simulink model "precompensationVSintegrator"  (R2018b)
settings: Solver=VariableStepAuto  StartTime=0.0  StopTime=2  RelTol=1e-3
values from neighbouring files (symbols this model uses):
  A = [-(bm*(n^2) + bg)/(Jm*(n^2) + Jg) Kt*n/(Jm*(n^2) + Jg) ... (first row only)    [DC_motor_geared_integral_discrete_sysid23.m]    (also in DC_motor_geared_lqr_discrete_sysid23.m; finalScript.m; finalScriptV2.m; precompensatorVSintegrator.m)
  B = [0 ... (first row only)    [DC_motor_geared_integral_discrete_sysid23.m]    (also in DC_motor_geared_lqr_discrete_sysid23.m; finalScript.m; finalScriptV2.m; precompensatorVSintegrator.m)
  Kc = lqr(sysd,Q,R)    [DC_motor_geared_lqr_discrete_sysid23.m]    (also in precompensatorVSintegrator.m = lqr(sysc,Q,R))
  Kdi = dlqr(Ad,Bd,Q,R)    [DC_motor_geared_integral_discrete_sysid23.m]    (also in finalScript.m; finalScriptV2.m)
  Nbar = rscale(sys_ss,Kc)    [DC_motor_geared_lqr_discrete_sysid23.m]    (also in precompensatorVSintegrator.m; rscale.m = Nu + K*Nx)
  Tsc = 1/20000    (= 5e-05)    [DC_motor_geared_integral_discrete_sysid23.m]    (also in DC_motor_geared_lqr_discrete_sysid23.m = 1e-05; finalScript.m; finalScriptV2.m = 0.001)
undefined symbols (not defined in the file or in its folder): DiscIntNeverNeededParam
libraries: pePwmGenerator x2
settings Model: Creator=Roberto  LastModifiedBy=Roberto

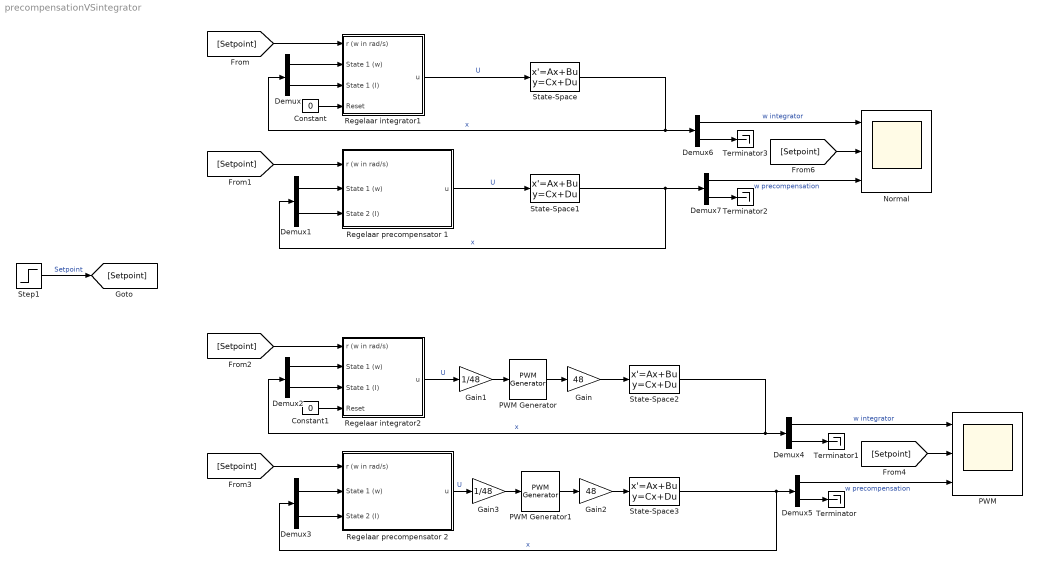
== system precompensationVSintegrator ==
  Constant : Constant  Value=0
  Constant1 : Constant  Value=0
  Demux{,1..7} (8 alike) : Demux  Outputs=2
  Gain : Gain  Gain=48
  Gain1 : Gain  Gain=1/48
  Gain2 : Gain  Gain=48
  Gain3 : Gain  Gain=1/48
  Normal : Scope  NumInputPorts=3
  PWM : Scope  NumInputPorts=3
  PWM Generator : pePwmGenerator/PWM Generator  CarrCount=Up  Tper=1/20000  Ts=1e-6
  PWM Generator1 : pePwmGenerator/PWM Generator  CarrCount=Up  Tper=1/20000  Ts=1e-6
  Regelaar integrator1 : Subsystem
  Regelaar integrator2 : Subsystem
  Regelaar precompensator 1 : Subsystem
  Regelaar precompensator 2 : Subsystem
  State-Space{,1..3} (4 alike) : StateSpace  A=A  B=B  C=eye(2)  D=[0; 0]  InitialCondition=0
  Step1 : Step  Time=0.1  After=25  SampleTime=0
  Terminator{,1..3} (4 alike) : Terminator
  wires:
  Regelaar integrator1/1(u) -> State-Space/1  "U"
  Step1/1 -> [Setpoint]  "Setpoint"
  [Setpoint] -> Regelaar integrator1/1(r (w in rad/s))
  [Setpoint] -> Regelaar precompensator 1/1(r (w in rad/s))
  Constant/1 -> Regelaar integrator1/4(Reset)
  Demux/1 -> Regelaar integrator1/2(State 1 (w))
  Demux/2 -> Regelaar integrator1/3(State 1 (I))
  Demux1/1 -> Regelaar precompensator 1/2(State 1 (w))
  Demux1/2 -> Regelaar precompensator 1/3(State 2 (I))
  Regelaar precompensator 1/1(u) -> State-Space1/1  "U"
  State-Space1/1 -> Demux7/1, Demux1/1  "x"
  State-Space/1 -> Demux/1, Demux6/1  "x"
  State-Space2/1 -> Demux4/1, Demux2/1  "x"
  Constant1/1 -> Regelaar integrator2/4(Reset)
  Demux3/2 -> Regelaar precompensator 2/3(State 2 (I))
  Demux2/1 -> Regelaar integrator2/2(State 1 (w))
  State-Space3/1 -> Demux5/1, Demux3/1  "x"
  [Setpoint] -> Regelaar precompensator 2/1(r (w in rad/s))
  Demux2/2 -> Regelaar integrator2/3(State 1 (I))
  [Setpoint] -> Regelaar integrator2/1(r (w in rad/s))
  Demux3/1 -> Regelaar precompensator 2/2(State 1 (w))
  Gain1/1 -> PWM Generator/1
  PWM Generator/1 -> Gain/1
  PWM Generator1/1 -> Gain2/1
  Gain3/1 -> PWM Generator1/1
  Regelaar precompensator 2/1(u) -> Gain3/1  "U"
  Regelaar integrator2/1(u) -> Gain1/1  "U"
  Gain/1 -> State-Space2/1
  Gain2/1 -> State-Space3/1
  [Setpoint] -> PWM/2
  Demux4/1 -> PWM/1  "w integrator"
  Demux5/1 -> PWM/3  "w precompensation"
  Demux5/2 -> Terminator/1
  Demux4/2 -> Terminator1/1
  [Setpoint] -> Normal/2
  Demux7/1 -> Normal/3  "w precompensation"
  Demux6/2 -> Terminator3/1
  Demux7/2 -> Terminator2/1
  Demux6/1 -> Normal/1  "w integrator"

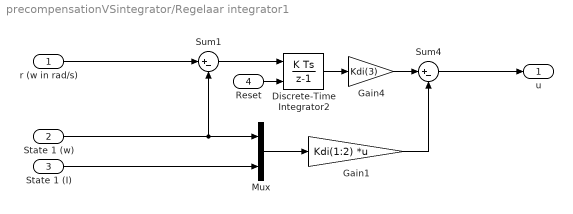
== system precompensationVSintegrator/Regelaar integrator1 ==
  r (w in rad/s) : Inport
  State 1 (w) : Inport  Port=2
  State 1 (I) : Inport  Port=3
  Reset : Inport  Port=4
  Discrete-Time Integrator2 : DiscreteIntegrator  gainval=1  ExternalReset=rising  SampleTime=Tsc  ICPrevOutput=DiscIntNeverNeededParam  ICPrevScaledInput=DiscIntNeverNeededParam
  Gain1 : Gain  Gain=Kdi(1:2)  Multiplication=Matrix(K*u)
  Gain4 : Gain  Gain=Kdi(3)
  Mux : Mux  Inputs=2
  Sum1 : Sum  Inputs=|+-
  Sum4 : Sum  Inputs=|+-
  u : Outport
  wires:
  r (w in rad/s)/1 -> Sum1/1
  State 1 (I)/1 -> Mux/2
  Mux/1 -> Gain1/1
  Gain1/1 -> Sum4/2
  Gain4/1 -> Sum4/1
  Sum4/1 -> u/1
  State 1 (w)/1 -> Mux/1, Sum1/2
  Sum1/1 -> Discrete-Time Integrator2/1
  Discrete-Time Integrator2/1 -> Gain4/1
  Reset/1 -> Discrete-Time Integrator2/2

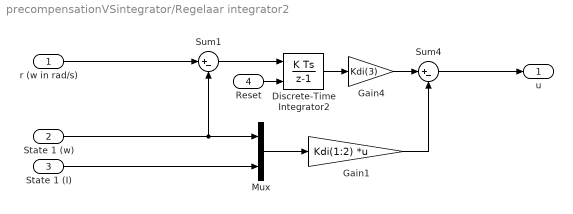
== system precompensationVSintegrator/Regelaar integrator2 ==
  r (w in rad/s) : Inport
  State 1 (w) : Inport  Port=2
  State 1 (I) : Inport  Port=3
  Reset : Inport  Port=4
  Discrete-Time Integrator2 : DiscreteIntegrator  gainval=1  ExternalReset=rising  SampleTime=Tsc  ICPrevOutput=DiscIntNeverNeededParam  ICPrevScaledInput=DiscIntNeverNeededParam
  Gain1 : Gain  Gain=Kdi(1:2)  Multiplication=Matrix(K*u)
  Gain4 : Gain  Gain=Kdi(3)
  Mux : Mux  Inputs=2
  Sum1 : Sum  Inputs=|+-
  Sum4 : Sum  Inputs=|+-
  u : Outport
  wires:
  r (w in rad/s)/1 -> Sum1/1
  State 1 (I)/1 -> Mux/2
  Mux/1 -> Gain1/1
  Gain1/1 -> Sum4/2
  Gain4/1 -> Sum4/1
  Sum4/1 -> u/1
  State 1 (w)/1 -> Mux/1, Sum1/2
  Sum1/1 -> Discrete-Time Integrator2/1
  Discrete-Time Integrator2/1 -> Gain4/1
  Reset/1 -> Discrete-Time Integrator2/2

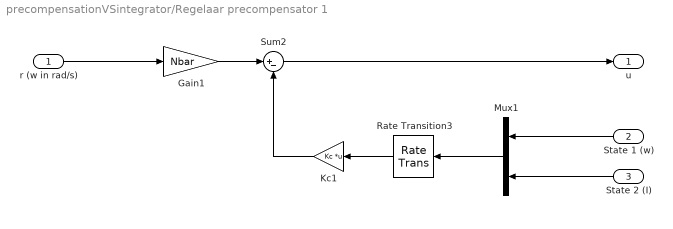
== system precompensationVSintegrator/Regelaar precompensator 1 ==
  r (w in rad/s) : Inport
  State 1 (w) : Inport  Port=2
  State 2 (I) : Inport  Port=3
  Gain1 : Gain  Gain=Nbar
  Kc1 : Gain  Gain=Kc  Multiplication=Matrix(K*u)
  Mux1 : Mux  Inputs=2
  Rate Transition3 : RateTransition  OutPortSampleTime=Tsc
  Sum2 : Sum  Inputs=|+-
  u : Outport
  wires:
  Mux1/1 -> Rate Transition3/1
  Rate Transition3/1 -> Kc1/1
  State 1 (w)/1 -> Mux1/1
  Kc1/1 -> Sum2/2
  Gain1/1 -> Sum2/1
  Sum2/1 -> u/1
  r (w in rad/s)/1 -> Gain1/1
  State 2 (I)/1 -> Mux1/2

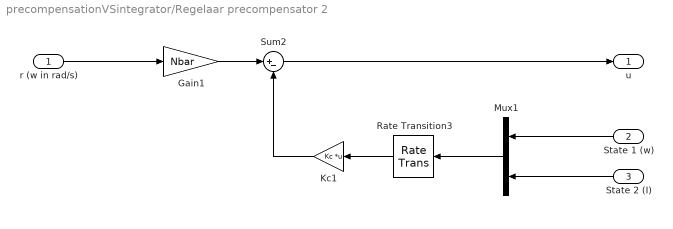
== system precompensationVSintegrator/Regelaar precompensator 2 ==
  r (w in rad/s) : Inport
  State 1 (w) : Inport  Port=2
  State 2 (I) : Inport  Port=3
  Gain1 : Gain  Gain=Nbar
  Kc1 : Gain  Gain=Kc  Multiplication=Matrix(K*u)
  Mux1 : Mux  Inputs=2
  Rate Transition3 : RateTransition  OutPortSampleTime=Tsc
  Sum2 : Sum  Inputs=|+-
  u : Outport
  wires:
  Mux1/1 -> Rate Transition3/1
  Rate Transition3/1 -> Kc1/1
  State 1 (w)/1 -> Mux1/1
  Kc1/1 -> Sum2/2
  Gain1/1 -> Sum2/1
  Sum2/1 -> u/1
  r (w in rad/s)/1 -> Gain1/1
  State 2 (I)/1 -> Mux1/2
